simulink subsystem "combining"  (R2021b)
settings: Solver=VariableStepAuto  StartTime=0.0  StopTime=10.0  RelTol=1e-3
undefined symbols (not defined in the file): antenna_num, sample_bitwidth, stream_num
settings Model: Creator=torha  LastModifiedBy=torha

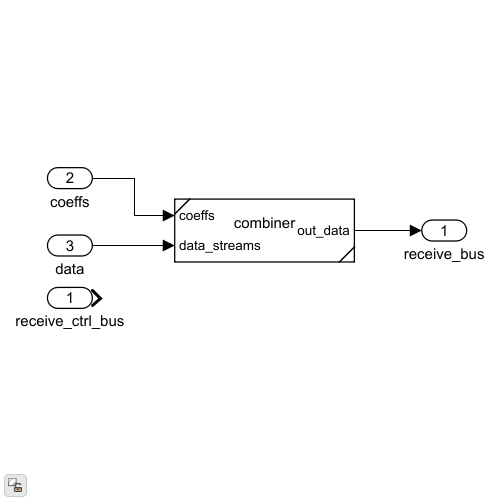
[thumbnail: Simulink's stored preview of the top-level diagram]
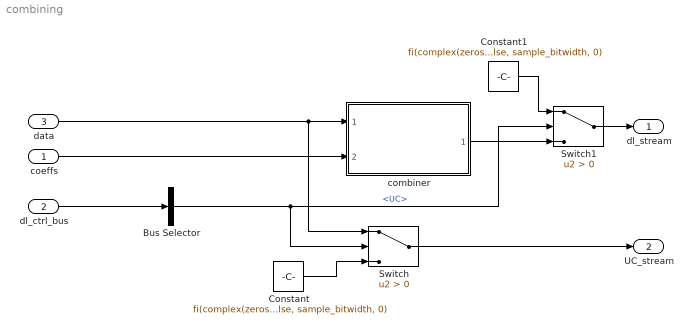
== system combining ==
  coeffs : Inport
  dl_ctrl_bus : Inport  Port=2
  data : Inport  Port=3
  Bus Selector : BusSelector  OutputSignals=UC
  Constant : Constant  Value=fi(complex(zeros(1, antenna_num)), false, sample_bitwidth, 0)
  Constant1 : Constant  Value=fi(complex(zeros(1, stream_num)), false, sample_bitwidth, 0)
  Switch : Switch  Criteria=u2 > Threshold
  Switch1 : Switch  Criteria=u2 > Threshold
  combiner : Subsystem  ReferencedSubsystem=combiner
  dl_stream : Outport
  UC_stream : Outport  Port=2
  wires:
  Switch1/1 -> dl_stream/1
  Constant1/1 -> Switch1/1
  Constant/1 -> Switch/3
  Bus Selector/1 -> Switch/2, Switch1/2  "<UC>"
  Switch/1 -> UC_stream/1
  dl_ctrl_bus/1 -> Bus Selector/1
  coeffs/1 -> combiner/2
  data/1 -> Switch/1, combiner/1
  combiner/1 -> Switch1/3
